simulink model "quad_model_simulink"  (R2018a)
settings: Solver=VariableStepAuto  StartTime=0.0  StopTime=20  RelTol=1e-3
values from neighbouring files (symbols this model uses):
  F = eye(4); F(2,1)=DT; F(4,3)=DT    [kalmantuner.m]    (also in quadcopter_estimation.m = sysD.A)
  G = zeros(4,4)    [kalmantuner.m]    (also in quadcopter_estimation.m = sysD.B)
  H = eye(4)    [kalmantuner.m]    (also in quadcopter_estimation.m = sysD.C)
  Kd = dlqr(sysD.A,sysD.B,Qc,Rc)    [quadcopter_estimation.m]
  P0 = 0.001*eye(4)    [quadcopter_estimation.m]
  Qdist = eye(4)    [kalmantuner.m]    (also in quadcopter_estimation.m = 2*eye(4); Qdist(2,2)=0.65; Qdist(4,4)=0.2)
  Rnoise = 100*diag([150,950,450,1000])    [kalmantuner.m]    (also in quadcopter_estimation.m = 100000000*Rnoise)
  sysC = ss(A,B,C,D)    [quadcopter_estimation.m]
  x0 = [deg2rad(7),deg2rad(-8),deg2rad(5),deg2rad(-7)]    [quadcopter_estimation.m]
undefined symbols (not defined in the file or in its folder): Discrete, Time
libraries: ctrlSharedLib x1, simulink x1
settings Model: Creator=h1liang  LastModifiedBy=h1liang

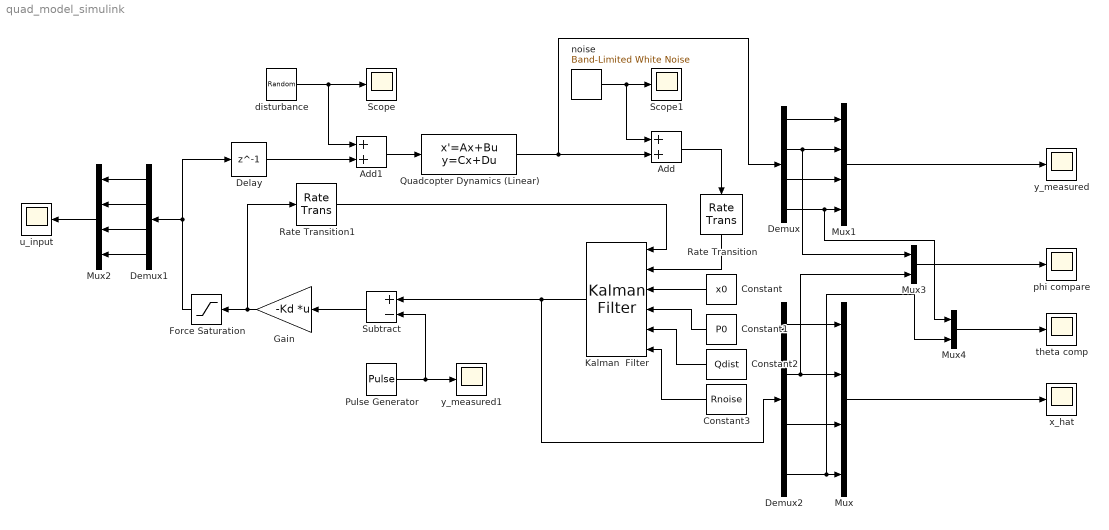
== system quad_model_simulink ==
  Add : Sum
  Add1 : Sum
  Constant : Constant  Value=x0
  Constant1 : Constant  Value=P0
  Constant2 : Constant  Value=Qdist  VectorParams1D=off
  Constant3 : Constant  Value=Rnoise  VectorParams1D=off
  Delay : Delay  DelayLength=1  InitialCondition=0
  Demux : Demux
  Demux1 : Demux
  Demux2 : Demux
  Force Saturation : Saturate  UpperLimit=8  LowerLimit=0
  Gain : Gain  Gain=-Kd  Multiplication=Matrix(K*u) (u vector)
  Kalman  Filter : ctrlSharedLib/Kalman Filter  TimeDomain=Discrete-Time  UseCurrentEstimator=on  ModelSource=Individual A, B, C, D matrices  ModelSourceVariable=ss(0.95,1,1,0,1)  A=F  B=G  C=H  D=0  NumberOfStates=1  NumberOfInputs=1  NumberOfOutputs=1  InitialEstimateSource=Input port  X0=0  P0=10  UseK=off  UseGH=off  NumberOfProcessNoiseInputs=1  G=G  TimeInvariantG=on  H=H  TimeInvariantH=on  Q=Qdist  TimeInvariantQ=off  R=Rnoise  TimeInvariantR=off  N=0  TimeInvariantN=on  AddInputPort=on  AddEnablePort=off  OutputEstimatedY=off  OutputP=off  Ts=0.01
      settings: SourceProductBaseCode=CT
  Mux : Mux
  Mux1 : Mux
  Mux2 : Mux
  Mux3 : Mux  Inputs=2
  Mux4 : Mux  Inputs=2
  Pulse Generator : DiscretePulseGenerator  PulseType=Time based  Amplitude=deg2rad(5)  Period=20  PulseWidth=50
  Quadcopter Dynamics (Linear) : StateSpace  A=sysC.A  B=sysC.B  C=sysC.C  D=sysC.D  InitialCondition=deg2rad([0,15,0,-10]')
  Rate Transition : RateTransition
  Rate Transition1 : RateTransition
  Scope : Scope
  Scope1 : Scope
  Subtract : Sum  Inputs=+-
  disturbance : UniformRandomNumber  SampleTime=0.2
  "noise " : simulink/Sources/Band-Limited White Noise  Cov=0.000001  Ts=0.01  seed=[23341]
  phi compare : Scope
  "theta comp " : Scope
  u_input : Scope
  x_hat : Scope
  y_measured : Scope
  y_measured1 : Scope
  wires:
  Demux2/1 -> Mux/1
  Demux2/3 -> Mux/3
  Mux/1 -> x_hat/1
  Demux/1 -> Mux1/1
  Demux/2 -> Mux1/2, Mux3/1
  Mux1/1 -> y_measured/1
  Demux1/2 -> Mux2/2
  Demux1/1 -> Mux2/1
  Demux1/3 -> Mux2/3
  Mux2/1 -> u_input/1
  Demux1/4 -> Mux2/4
  Quadcopter Dynamics (Linear)/1 -> Add/2, Demux/1
  Add/1 -> Rate Transition/1
  Add1/1 -> Quadcopter Dynamics (Linear)/1
  Mux3/1 -> phi compare/1
  Mux4/1 -> "theta comp "/1
  Demux2/4 -> Mux4/2, Mux/4
  Demux2/2 -> Mux/2, Mux3/2
  Force Saturation/1 -> Delay/1, Demux1/1
  Pulse Generator/1 -> y_measured1/1, Subtract/2
  "noise "/1 -> Add/1, Scope1/1
  disturbance/1 -> Add1/1, Scope/1
  Gain/1 -> Rate Transition1/1, Force Saturation/1
  Kalman  Filter/1 -> Subtract/1, Demux2/1
  Constant/1 -> Kalman  Filter/3
  Rate Transition/1 -> Kalman  Filter/2
  Subtract/1 -> Gain/1
  Rate Transition1/1 -> Kalman  Filter/1
  Delay/1 -> Add1/2
  Demux/3 -> Mux1/3
  Demux/4 -> Mux4/1, Mux1/4
  Constant2/1 -> Kalman  Filter/5
  Constant3/1 -> Kalman  Filter/6
  Constant1/1 -> Kalman  Filter/4
